simulink model "wyz_M"  (R2022a)
settings: Solver=VariableStepAuto  StartTime=0.0  StopTime=60  RelTol=1e-3
undefined symbols (not defined in the file): A, b, c
settings Model: Creator=andrzej  LastModifiedBy=andrzej
settings DataIOCC: SaveFormat=Array  ReturnWorkspaceOutputs=off

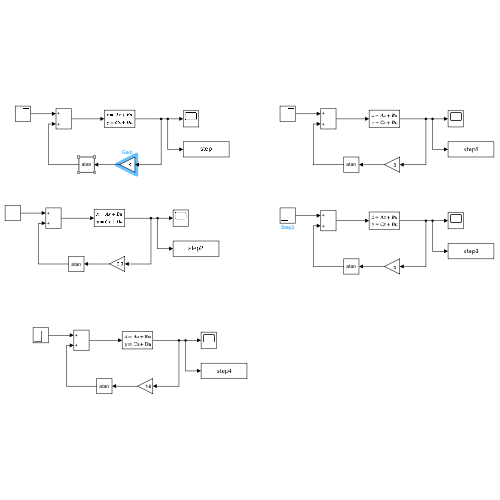
[thumbnail: Simulink's stored preview of the top-level diagram]
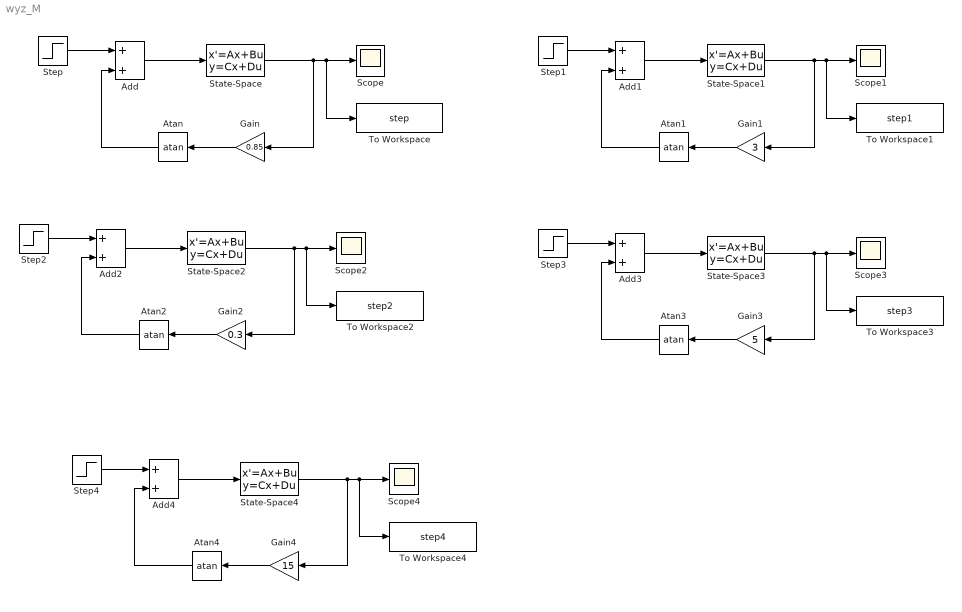
== system wyz_M ==
  Add{,1..4} (5 alike) : Sum
  Atan{,1..4} (5 alike) : Trigonometry  Operator=atan
  Gain : Gain  Gain=0.85
  Gain1 : Gain  Gain=3
  Gain2 : Gain  Gain=0.3
  Gain3 : Gain  Gain=5
  Gain4 : Gain  Gain=15
  Scope{,1..4} (5 alike) : Scope
  State-Space{,1..4} (5 alike) : StateSpace  A=A  B=b  C=c  D=[0]  InitialCondition=0
  Step{,1..4} (5 alike) : Step  SampleTime=0
  To Workspace : ToWorkspace  VariableName=step  SampleTime=-1
      settings: Save2DSignal=2-D array (concatenate along first dimension)
  To Workspace1 : ToWorkspace  VariableName=step1  SampleTime=-1
      settings: Save2DSignal=2-D array (concatenate along first dimension)
  To Workspace2 : ToWorkspace  VariableName=step2  SampleTime=-1
      settings: Save2DSignal=2-D array (concatenate along first dimension)
  To Workspace3 : ToWorkspace  VariableName=step3  SampleTime=-1
      settings: Save2DSignal=2-D array (concatenate along first dimension)
  To Workspace4 : ToWorkspace  VariableName=step4  SampleTime=-1
      settings: Save2DSignal=2-D array (concatenate along first dimension)
  wires:
  State-Space/1 -> Gain/1, To Workspace/1, Scope/1
  Gain/1 -> Atan/1
  Add/1 -> State-Space/1
  Step/1 -> Add/1
  Atan/1 -> Add/2
  State-Space1/1 -> Gain1/1, To Workspace1/1, Scope1/1
  Gain1/1 -> Atan1/1
  Step1/1 -> Add1/1
  Add1/1 -> State-Space1/1
  Atan1/1 -> Add1/2
  State-Space2/1 -> Gain2/1, To Workspace2/1, Scope2/1
  Gain2/1 -> Atan2/1
  Step2/1 -> Add2/1
  Add2/1 -> State-Space2/1
  Atan2/1 -> Add2/2
  State-Space3/1 -> Gain3/1, To Workspace3/1, Scope3/1
  Gain3/1 -> Atan3/1
  Step3/1 -> Add3/1
  Add3/1 -> State-Space3/1
  Atan3/1 -> Add3/2
  State-Space4/1 -> Gain4/1, To Workspace4/1, Scope4/1
  Gain4/1 -> Atan4/1
  Step4/1 -> Add4/1
  Add4/1 -> State-Space4/1
  Atan4/1 -> Add4/2
